simulink model "Parallel_n49"  (R2012b)
settings: Solver=VariableStepDiscrete  StartTime=0.0  StopTime=TotalIterations  RelTol=1e-3
values from neighbouring files (symbols this model uses):
  bp = 12    [ConfigValidate.m]
  bpSNMemory = bp    (= 12)    [ConfigValidate.m]
  IterationsOrdering = 4000    [ConfigValidate.m]
  MaxCoordDistance = (abs(max(wx) - min(wx))+abs(max(wy) - min(wy)))^2    [ConfigValidate.m]
  N_limit = 0.01    [ConfigValidate.m]
  nBits = 9    [ConfigValidate.m]
  nBitsNSmemories = (ceil(log2(TotalIterations)))    [ConfigValidate.m]
  S_limit = 1    [ConfigValidate.m]
  SourceNodes = 2000    [ConfigValidate.m]
  ts = 1    [ConfigValidate.m]
  w1 = rand(1,Neurons)    [ConfigValidate.m]
  w2 = rand(1,Neurons)    [ConfigValidate.m]
  wx = zeros(1,Neurons)    [ConfigValidate.m]
  wy = zeros(1,Neurons)    [ConfigValidate.m]
  x1 = rand(SourceNodes,1)    [ConfigValidate.m]
  x2 = rand(SourceNodes,1)    [ConfigValidate.m]
libraries: xbsIndex_r4 x4147, dspsrcs4 x2, dspstat3 x2
(part 1 of 19)
settings Model: Creator=Leonardo  LastModifiedBy=leona

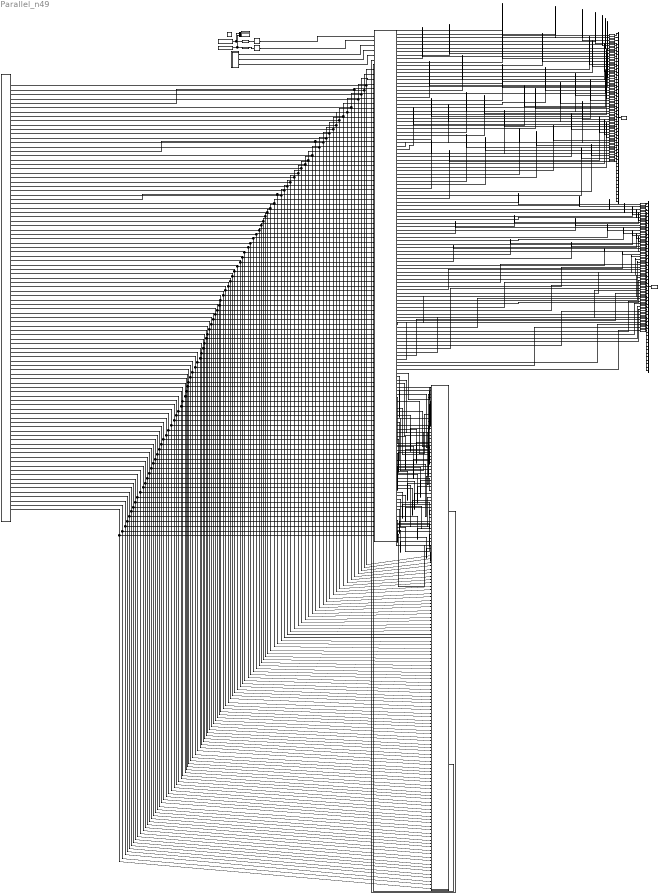
== system Parallel_n49 ==
  " System Generator" : xbsIndex_r4/ System Generator  Tag=genX  xilinxfamily=virtex6  part=xc6vlx240t  speed=-1  package=ff1156  synthesis_tool=XST  clock_wrapper=Clock Enables  directory=./n49d2nt  proj_type=Project Navigator  Synth_file=XST Defaults  Impl_file=ISE Defaults  testbench=off  simulink_period=ts  sysclk_period=10  dcm_input_clock_period=10  incr_netlist=off  trim_vbits=Everywhere in SubSystem  dbl_ovrd=According to Block Masks  core_generation=According to Block Masks  run_coregen=off  deprecated_control=off  eval_field=0  block_type=sysgen
  Coordinates : Subsystem
  Display2 : Display
  Gateway Out{1,3..48,53,65..75,77..107,109,113,120,126..128} (96 alike) : xbsIndex_r4/Gateway Out  inherit_from_input=off  hdl_port=off  timing_constraint=None  locs_specified=off  LOCs={}  UseAsDAC=off  DACChannel='1'  block_type=gatewayout
  Gateway Out2 : xbsIndex_r4/Gateway Out  inherit_from_input=off  hdl_port=on  timing_constraint=None  locs_specified=off  LOCs={}  UseAsDAC=off  DACChannel='1'  block_type=gatewayout
  Gateway Out76 : xbsIndex_r4/Gateway Out  inherit_from_input=off  hdl_port=on  timing_constraint=None  locs_specified=off  LOCs={}  UseAsDAC=off  DACChannel='1'  block_type=gatewayout
  Mux1 : Mux  Inputs=49
  Mux3 : Mux  Inputs=2
  Mux5 : Mux  Inputs=49
  Neurons : Subsystem
  Signal From Workspace : dspsrcs4/Signal From Workspace  X=x1(1:SourceNodes)  Ts=ts  nsamps=1  OutputAfterFinalValue=Cyclic repetition  ignoreOrWarnInputAndFrameLengths=off
  Signal From Workspace1 : dspsrcs4/Signal From Workspace  X=x2(1:SourceNodes)  Ts=ts  nsamps=1  OutputAfterFinalValue=Cyclic repetition  ignoreOrWarnInputAndFrameLengths=off
  TimeSeries_Functions : Subsystem
  To Workspace : ToWorkspace  VariableName=w1_histH  SampleTime=ts
  To Workspace1 : ToWorkspace  VariableName=w2_histH  SampleTime=ts
  WiningNeuronFinder1 : Subsystem
  delay_vX11 : xbsIndex_r4/Register  init=x1(1)  rst=off  en=off  dbl_ovrd=off  block_type=register
  delay_vX12 : xbsIndex_r4/Register  init=x2(1)  rst=off  en=off  dbl_ovrd=off  block_type=register
  "vX11_in " : xbsIndex_r4/Gateway In  gui_display_data_type=Fixed-point  arith_type="Signed  (2's comp)"  n_bits=nb  bin_pt=bp  preci_type=Single  exp_width=8  frac_width=24  quantization="Round  (unbiased: +/- Inf)"  overflow=Saturate  period=ts  dbl_ovrd=off  timing_constraint=None  locs_specified=off  LOCs={}  UseAsADC=off  ADCChannel='1'  inherit_from_input=off  hdl_port=on  block_type=gatewayin
  vX12_in : xbsIndex_r4/Gateway In  gui_display_data_type=Fixed-point  arith_type="Signed  (2's comp)"  n_bits=nb  bin_pt=bp  preci_type=Single  exp_width=8  frac_width=24  quantization="Round  (unbiased: +/- Inf)"  overflow=Saturate  period=ts  dbl_ovrd=off  timing_constraint=None  locs_specified=off  LOCs={}  UseAsADC=off  ADCChannel='1'  inherit_from_input=off  hdl_port=on  block_type=gatewayin
  wires:
  Signal From Workspace/1 -> Mux3/1, "vX11_in "/1
  Signal From Workspace1/1 -> Mux3/2, vX12_in/1
  Mux3/1 -> Display2/1
  vX12_in/1 -> delay_vX12/1
  delay_vX12/1 -> Neurons/2(vX12)
  TimeSeries_Functions/1(S) -> Neurons/3(S)
  TimeSeries_Functions/2(N) -> Neurons/4(N)
  TimeSeries_Functions/3(MemControl) -> Neurons/5(memControl)
  Mux5/1 -> To Workspace/1
  "vX11_in "/1 -> delay_vX11/1
  delay_vX11/1 -> Neurons/1(vX11)
  Neurons/34(w1n34) -> Gateway Out27/1
  Neurons/35(w1n35) -> Gateway Out26/1
  Neurons/31(w1n31) -> Gateway Out35/1
  Neurons/33(w1n33) -> Gateway Out36/1
  Neurons/32(w1n32) -> Gateway Out34/1
  Neurons/40(w1n40) -> Gateway Out44/1
  Neurons/45(w1n45) -> Gateway Out48/1
  Neurons/36(w1n36) -> Gateway Out28/1
  Neurons/44(w1n44) -> Gateway Out46/1
  Neurons/39(w1n39) -> Gateway Out42/1
  Neurons/43(w1n43) -> Gateway Out47/1
  Neurons/42(w1n42) -> Gateway Out45/1
  Neurons/37(w1n37) -> Gateway Out41/1
  Neurons/38(w1n38) -> Gateway Out37/1
  Neurons/41(w1n41) -> Gateway Out43/1
  Neurons/27(w1n27) -> Gateway Out30/1
  Neurons/26(w1n26) -> Gateway Out25/1
  Neurons/29(w1n29) -> Gateway Out31/1
  Neurons/28(w1n28) -> Gateway Out32/1
  Neurons/30(w1n30) -> Gateway Out33/1
  Neurons/6(w1n6) -> Gateway Out6/1
  Neurons/9(w1n9) -> Gateway Out9/1
  Neurons/10(w1n10) -> Gateway Out11/1
  Neurons/1(w1n1) -> Gateway Out2/1
  Neurons/2(w1n2) -> Gateway Out1/1
  Neurons/3(w1n3) -> Gateway Out3/1
  Neurons/4(w1n4) -> Gateway Out5/1
  Neurons/5(w1n5) -> Gateway Out4/1
  Neurons/7(w1n7) -> Gateway Out8/1
  Neurons/8(w1n8) -> Gateway Out7/1
  Neurons/23(w1n23) -> Gateway Out14/1
  Neurons/12(w1n12) -> Gateway Out12/1
  Neurons/11(w1n11) -> Gateway Out10/1
  Neurons/14(w1n14) -> Gateway Out13/1
  Neurons/19(w1n19) -> Gateway Out23/1
  Neurons/24(w1n24) -> Gateway Out16/1
  Neurons/13(w1n13) -> Gateway Out17/1
  Neurons/15(w1n15) -> Gateway Out18/1
  Neurons/18(w1n18) -> Gateway Out21/1
  Neurons/17(w1n17) -> Gateway Out19/1
  Neurons/20(w1n20) -> Gateway Out22/1
  Neurons/22(w1n22) -> Gateway Out15/1
  Neurons/25(w1n25) -> Gateway Out29/1
  Neurons/16(w1n16) -> Gateway Out20/1
  Neurons/21(w1n21) -> Gateway Out24/1
  Neurons/48(w1n48) -> Gateway Out40/1
  Neurons/46(w1n46) -> Gateway Out39/1
  Neurons/49(w1n49) -> Gateway Out53/1
  Neurons/47(w1n47) -> Gateway Out38/1
  Mux1/1 -> To Workspace1/1
  Neurons/70(w2n21) -> Gateway Out81/1
  Neurons/72(w2n23) -> Gateway Out70/1
  Neurons/71(w2n22) -> Gateway Out71/1
  Neurons/74(w2n25) -> Gateway Out86/1
  Neurons/73(w2n24) -> Gateway Out72/1
  Neurons/60(w2n11) -> Gateway Out66/1
  Neurons/63(w2n14) -> Gateway Out69/1
  Neurons/62(w2n13) -> Gateway Out73/1
  Neurons/64(w2n15) -> Gateway Out74/1
  Neurons/61(w2n12) -> Gateway Out68/1
  Neurons/54(w2n5) -> Gateway Out98/1
  Neurons/85(w2n36) -> Gateway Out85/1
  Neurons/88(w2n39) -> Gateway Out101/1
  Neurons/89(w2n40) -> Gateway Out103/1
  Neurons/86(w2n37) -> Gateway Out100/1
  Neurons/87(w2n38) -> Gateway Out95/1
  Neurons/94(w2n45) -> Gateway Out107/1
  Neurons/93(w2n44) -> Gateway Out105/1
  Neurons/92(w2n43) -> Gateway Out106/1
  Neurons/90(w2n41) -> Gateway Out102/1
  Neurons/91(w2n42) -> Gateway Out104/1
  Neurons/65(w2n16) -> Gateway Out77/1
  Neurons/68(w2n19) -> Gateway Out80/1
  Neurons/67(w2n18) -> Gateway Out78/1
  Neurons/66(w2n17) -> Gateway Out75/1
  Neurons/69(w2n20) -> Gateway Out79/1
  Neurons/55(w2n6) -> Gateway Out120/1
  Neurons/56(w2n7) -> Gateway Out127/1
  Neurons/59(w2n10) -> Gateway Out67/1
  Neurons/57(w2n8) -> Gateway Out126/1
  Neurons/58(w2n9) -> Gateway Out128/1
  Neurons/75(w2n26) -> Gateway Out82/1
  Neurons/78(w2n29) -> Gateway Out89/1
  Neurons/79(w2n30) -> Gateway Out91/1
  Neurons/76(w2n27) -> Gateway Out88/1
  Neurons/77(w2n28) -> Gateway Out90/1
  Neurons/52(w2n3) -> Gateway Out87/1
  Neurons/95(w2n46) -> Gateway Out97/1
  Neurons/97(w2n48) -> Gateway Out99/1
  Neurons/96(w2n47) -> Gateway Out96/1
  Neurons/98(w2n49) -> Gateway Out113/1
  Neurons/51(w2n2) -> Gateway Out65/1
  Neurons/50(w2n1) -> Gateway Out76/1
  Neurons/80(w2n31) -> Gateway Out93/1
  Neurons/81(w2n32) -> Gateway Out92/1
  Neurons/82(w2n33) -> Gateway Out94/1
  Neurons/84(w2n35) -> Gateway Out83/1
  Neurons/83(w2n34) -> Gateway Out84/1
  Neurons/53(w2n4) -> Gateway Out109/1
  Gateway Out2/1 -> Mux5/1
  Gateway Out1/1 -> Mux5/2
  Gateway Out3/1 -> Mux5/3
  Gateway Out5/1 -> Mux5/4
  Gateway Out6/1 -> Mux5/6
  Gateway Out4/1 -> Mux5/5
  Gateway Out8/1 -> Mux5/7
  Gateway Out10/1 -> Mux5/11
  Gateway Out9/1 -> Mux5/9
  Gateway Out7/1 -> Mux5/8
  Gateway Out11/1 -> Mux5/10
  Gateway Out12/1 -> Mux5/12
  Gateway Out13/1 -> Mux5/14
  Gateway Out22/1 -> Mux5/20
  Gateway Out17/1 -> Mux5/13
  Gateway Out20/1 -> Mux5/16
  Gateway Out14/1 -> Mux5/23
  Gateway Out15/1 -> Mux5/22
  Gateway Out16/1 -> Mux5/24
  Gateway Out19/1 -> Mux5/17
  Gateway Out18/1 -> Mux5/15
  Gateway Out21/1 -> Mux5/18
  Gateway Out23/1 -> Mux5/19
  Gateway Out24/1 -> Mux5/21
  Gateway Out25/1 -> Mux5/26
  Gateway Out27/1 -> Mux5/34
  Gateway Out26/1 -> Mux5/35
  Gateway Out28/1 -> Mux5/36
  Gateway Out36/1 -> Mux5/33
  Gateway Out30/1 -> Mux5/27
  Gateway Out32/1 -> Mux5/28
  Gateway Out29/1 -> Mux5/25
  Gateway Out35/1 -> Mux5/31
  Gateway Out31/1 -> Mux5/29
  Gateway Out34/1 -> Mux5/32
  Gateway Out33/1 -> Mux5/30
  Gateway Out45/1 -> Mux5/42
  Gateway Out43/1 -> Mux5/41
  Gateway Out44/1 -> Mux5/40
  Gateway Out46/1 -> Mux5/44
  Gateway Out39/1 -> Mux5/46
  Gateway Out41/1 -> Mux5/37
  Gateway Out40/1 -> Mux5/48
  Gateway Out38/1 -> Mux5/47
  Gateway Out42/1 -> Mux5/39
  Gateway Out37/1 -> Mux5/38
  Gateway Out48/1 -> Mux5/45
  Gateway Out47/1 -> Mux5/43
  Gateway Out53/1 -> Mux5/49
  Gateway Out66/1 -> Mux1/11
  Gateway Out69/1 -> Mux1/14
  Gateway Out67/1 -> Mux1/10
  Gateway Out70/1 -> Mux1/23
  Gateway Out68/1 -> Mux1/12
  Gateway Out73/1 -> Mux1/13
  Gateway Out72/1 -> Mux1/24
  Gateway Out75/1 -> Mux1/17
  Gateway Out71/1 -> Mux1/22
  Gateway Out74/1 -> Mux1/15
  Gateway Out79/1 -> Mux1/20
  Gateway Out80/1 -> Mux1/19
  Gateway Out76/1 -> Mux1/1
  Gateway Out77/1 -> Mux1/16
  Gateway Out78/1 -> Mux1/18
  Gateway Out84/1 -> Mux1/34
  Gateway Out85/1 -> Mux1/36
  Gateway Out82/1 -> Mux1/26
  Gateway Out81/1 -> Mux1/21
  Gateway Out83/1 -> Mux1/35
  Gateway Out88/1 -> Mux1/27
  Gateway Out90/1 -> Mux1/28
  Gateway Out89/1 -> Mux1/29
  Gateway Out86/1 -> Mux1/25
  Gateway Out87/1 -> Mux1/3
  Gateway Out92/1 -> Mux1/32
  Gateway Out93/1 -> Mux1/31
  Gateway Out94/1 -> Mux1/33
  Gateway Out91/1 -> Mux1/30
  Gateway Out95/1 -> Mux1/38
  Gateway Out96/1 -> Mux1/47
  Gateway Out98/1 -> Mux1/5
  Gateway Out97/1 -> Mux1/46
  Gateway Out99/1 -> Mux1/48
  Gateway Out101/1 -> Mux1/39
  Gateway Out100/1 -> Mux1/37
  Gateway Out65/1 -> Mux1/2
  Gateway Out102/1 -> Mux1/41
  Gateway Out113/1 -> Mux1/49
  Gateway Out106/1 -> Mux1/43
  Gateway Out105/1 -> Mux1/44
  Gateway Out104/1 -> Mux1/42
  Gateway Out109/1 -> Mux1/4
  Gateway Out107/1 -> Mux1/45
  Gateway Out103/1 -> Mux1/40
  Gateway Out127/1 -> Mux1/7
  Gateway Out128/1 -> Mux1/9
  Gateway Out120/1 -> Mux1/6
  Gateway Out126/1 -> Mux1/8
  Neurons/109(dist_n11) -> WiningNeuronFinder1/11(dist_k11)
  Neurons/113(dist_n15) -> WiningNeuronFinder1/15(dist_k15)
  Neurons/112(dist_n14) -> WiningNeuronFinder1/14(dist_k14)
  Neurons/110(dist_n12) -> WiningNeuronFinder1/12(dist_k12)
  Neurons/111(dist_n13) -> WiningNeuronFinder1/13(dist_k13)
  Neurons/120(dist_n22) -> WiningNeuronFinder1/22(dist_k22)
  Neurons/123(dist_n25) -> WiningNeuronFinder1/25(dist_k25)
  Neurons/122(dist_n24) -> WiningNeuronFinder1/24(dist_k24)
  Neurons/121(dist_n23) -> WiningNeuronFinder1/23(dist_k23)
  Neurons/119(dist_n21) -> WiningNeuronFinder1/21(dist_k21)
  Neurons/114(dist_n16) -> WiningNeuronFinder1/16(dist_k16)
  Neurons/115(dist_n17) -> WiningNeuronFinder1/17(dist_k17)
  Neurons/118(dist_n20) -> WiningNeuronFinder1/20(dist_k20)
  Neurons/117(dist_n19) -> WiningNeuronFinder1/19(dist_k19)
  Neurons/116(dist_n18) -> WiningNeuronFinder1/18(dist_k18)
  Neurons/99(dist_n1) -> WiningNeuronFinder1/1(dist_k1)
  Neurons/139(dist_n41) -> WiningNeuronFinder1/41(dist_k41)
  Neurons/142(dist_n44) -> WiningNeuronFinder1/44(dist_k44)
  Neurons/141(dist_n43) -> WiningNeuronFinder1/43(dist_k43)
  Neurons/143(dist_n45) -> WiningNeuronFinder1/45(dist_k45)
  Neurons/140(dist_n42) -> WiningNeuronFinder1/42(dist_k42)
  Neurons/145(dist_n47) -> WiningNeuronFinder1/47(dist_k47)
  Neurons/144(dist_n46) -> WiningNeuronFinder1/46(dist_k46)
  Neurons/146(dist_n48) -> WiningNeuronFinder1/48(dist_k48)
  Neurons/147(dist_n49) -> WiningNeuronFinder1/49(dist_k49)
  Neurons/101(dist_n3) -> WiningNeuronFinder1/3(dist_k3)
  Neurons/102(dist_n4) -> WiningNeuronFinder1/4(dist_k4)
  Neurons/125(dist_n27) -> WiningNeuronFinder1/27(dist_k27)
  Neurons/126(dist_n28) -> WiningNeuronFinder1/28(dist_k28)
  Neurons/127(dist_n29) -> WiningNeuronFinder1/29(dist_k29)
  Neurons/128(dist_n30) -> WiningNeuronFinder1/30(dist_k30)
  Neurons/124(dist_n26) -> WiningNeuronFinder1/26(dist_k26)
  Neurons/100(dist_n2) -> WiningNeuronFinder1/2(dist_k2)
  Neurons/129(dist_n31) -> WiningNeuronFinder1/31(dist_k31)
  Neurons/133(dist_n35) -> WiningNeuronFinder1/35(dist_k35)
  Neurons/131(dist_n33) -> WiningNeuronFinder1/33(dist_k33)
  Neurons/130(dist_n32) -> WiningNeuronFinder1/32(dist_k32)
  Neurons/132(dist_n34) -> WiningNeuronFinder1/34(dist_k34)
  Neurons/138(dist_n40) -> WiningNeuronFinder1/40(dist_k40)
  Neurons/136(dist_n38) -> WiningNeuronFinder1/38(dist_k38)
  Neurons/135(dist_n37) -> WiningNeuronFinder1/37(dist_k37)
  Neurons/134(dist_n36) -> WiningNeuronFinder1/36(dist_k36)
  Neurons/137(dist_n39) -> WiningNeuronFinder1/39(dist_k39)
  Neurons/103(dist_n5) -> WiningNeuronFinder1/5(dist_k5)
  Neurons/108(dist_n10) -> WiningNeuronFinder1/10(dist_k10)
  Neurons/107(dist_n9) -> WiningNeuronFinder1/9(dist_k9)
  Neurons/104(dist_n6) -> WiningNeuronFinder1/6(dist_k6)
  Neurons/106(dist_n8) -> WiningNeuronFinder1/8(dist_k8)
  Neurons/105(dist_n7) -> WiningNeuronFinder1/7(dist_k7)
  WiningNeuronFinder1/1(WinningNeuron_wx) -> Neurons/6(wx_win)
  WiningNeuronFinder1/2(WinningNeuron_wy) -> Neurons/7(wy_win)
  Coordinates/98(wy49) -> WiningNeuronFinder1/147(wy_49), Neurons/105(wy49)
  Coordinates/97(wx49) -> WiningNeuronFinder1/146(wx_49), Neurons/104(wx49)
  Coordinates/96(wy48) -> WiningNeuronFinder1/145(wy_48), Neurons/103(wy48)
  Coordinates/95(wx48) -> WiningNeuronFinder1/144(wx_48), Neurons/102(wx48)
  Coordinates/93(wx47) -> WiningNeuronFinder1/142(wx_47), Neurons/100(wx47)
  Coordinates/92(wy46) -> WiningNeuronFinder1/141(wy_46), Neurons/99(wy46)
  Coordinates/91(wx46) -> WiningNeuronFinder1/140(wx_46), Neurons/98(wx46)
  Coordinates/90(wy45) -> WiningNeuronFinder1/139(wy_45), Neurons/97(wy45)
  Coordinates/88(wy44) -> WiningNeuronFinder1/137(wy_44), Neurons/95(wy44)
  Coordinates/87(wx44) -> WiningNeuronFinder1/136(wx_44), Neurons/94(wx44)
  Coordinates/86(wy43) -> WiningNeuronFinder1/135(wy_43), Neurons/93(wy43)
  Coordinates/85(wx43) -> WiningNeuronFinder1/134(wx_43), Neurons/92(wx43)
  Coordinates/84(wy42) -> WiningNeuronFinder1/133(wy_42), Neurons/91(wy42)
  Coordinates/83(wx42) -> WiningNeuronFinder1/132(wx_42), Neurons/90(wx42)
  Coordinates/81(wx41) -> WiningNeuronFinder1/130(wx_41), Neurons/88(wx41)
  Coordinates/80(wy40) -> WiningNeuronFinder1/129(wy_40), Neurons/87(wy40)
  Coordinates/79(wx40) -> WiningNeuronFinder1/128(wx_40), Neurons/86(wx40)
  Coordinates/78(wy39) -> WiningNeuronFinder1/127(wy_39), Neurons/85(wy39)
  Coordinates/77(wx39) -> WiningNeuronFinder1/126(wx_39), Neurons/84(wx39)
  Coordinates/76(wy38) -> WiningNeuronFinder1/125(wy_38), Neurons/83(wy38)
  Coordinates/75(wx38) -> WiningNeuronFinder1/124(wx_38), Neurons/82(wx38)
  Coordinates/74(wy37) -> WiningNeuronFinder1/123(wy_37), Neurons/81(wy37)
  Coordinates/73(wx37) -> WiningNeuronFinder1/122(wx_37), Neurons/80(wx37)
  Coordinates/72(wy36) -> WiningNeuronFinder1/121(wy_36), Neurons/79(wy36)
  Coordinates/71(wx36) -> WiningNeuronFinder1/120(wx_36), Neurons/78(wx36)
  Coordinates/70(wy35) -> WiningNeuronFinder1/119(wy_35), Neurons/77(wy35)
  Coordinates/69(wx35) -> WiningNeuronFinder1/118(wx_35), Neurons/76(wx35)
  Coordinates/68(wy34) -> WiningNeuronFinder1/117(wy_34), Neurons/75(wy34)
  Coordinates/67(wx34) -> WiningNeuronFinder1/116(wx_34), Neurons/74(wx34)
  Coordinates/66(wy33) -> WiningNeuronFinder1/115(wy_33), Neurons/73(wy33)
  Coordinates/65(wx33) -> WiningNeuronFinder1/114(wx_33), Neurons/72(wx33)
  Coordinates/63(wx32) -> WiningNeuronFinder1/112(wx_32), Neurons/70(wx32)
  Coordinates/62(wy31) -> WiningNeuronFinder1/111(wy_31), Neurons/69(wy31)
  Coordinates/61(wx31) -> WiningNeuronFinder1/110(wx_31), Neurons/68(wx31)
  Coordinates/59(wx30) -> WiningNeuronFinder1/108(wx_30), Neurons/66(wx30)
  Coordinates/58(wy29) -> WiningNeuronFinder1/107(wy_29), Neurons/65(wy29)
  Coordinates/57(wx29) -> WiningNeuronFinder1/106(wx_29), Neurons/64(wx29)
  Coordinates/56(wy28) -> WiningNeuronFinder1/105(wy_28), Neurons/63(wy28)
  Coordinates/54(wy27) -> WiningNeuronFinder1/103(wy_27), Neurons/61(wy27)
  Coordinates/53(wx27) -> WiningNeuronFinder1/102(wx_27), Neurons/60(wx27)
  Coordinates/52(wy26) -> WiningNeuronFinder1/101(wy_26), Neurons/59(wy26)
  Coordinates/51(wx26) -> WiningNeuronFinder1/100(wx_26), Neurons/58(wx26)
  Coordinates/50(wy25) -> WiningNeuronFinder1/99(wy_25), Neurons/57(wy25)
  Coordinates/49(wx25) -> WiningNeuronFinder1/98(wx_25), Neurons/56(wx25)
  Coordinates/48(wy24) -> WiningNeuronFinder1/97(wy_24), Neurons/55(wy24)
  Coordinates/47(wx24) -> WiningNeuronFinder1/96(wx_24), Neurons/54(wx24)
  Coordinates/46(wy23) -> WiningNeuronFinder1/95(wy_23), Neurons/53(wy23)
  Coordinates/45(wx23) -> WiningNeuronFinder1/94(wx_23), Neurons/52(wx23)
  Coordinates/43(wx22) -> WiningNeuronFinder1/92(wx_22), Neurons/50(wx22)
  Coordinates/42(wy21) -> WiningNeuronFinder1/91(wy_21), Neurons/49(wy21)
  Coordinates/41(wx21) -> WiningNeuronFinder1/90(wx_21), Neurons/48(wx21)
  Coordinates/40(wy20) -> WiningNeuronFinder1/89(wy_20), Neurons/47(wy20)
  Coordinates/39(wx20) -> WiningNeuronFinder1/88(wx_20), Neurons/46(wx20)
  Coordinates/38(wy19) -> WiningNeuronFinder1/87(wy_19), Neurons/45(wy19)
  Coordinates/37(wx19) -> WiningNeuronFinder1/86(wx_19), Neurons/44(wx19)
  Coordinates/36(wy18) -> WiningNeuronFinder1/85(wy_18), Neurons/43(wy18)
  Coordinates/35(wx18) -> WiningNeuronFinder1/84(wx_18), Neurons/42(wx18)
  Coordinates/34(wy17) -> WiningNeuronFinder1/83(wy_17), Neurons/41(wy17)
  Coordinates/32(wy16) -> WiningNeuronFinder1/81(wy_16), Neurons/39(wy16)
  Coordinates/31(wx16) -> WiningNeuronFinder1/80(wx_16), Neurons/38(wx16)
  Coordinates/30(wy15) -> WiningNeuronFinder1/79(wy_15), Neurons/37(wy15)
  Coordinates/29(wx15) -> WiningNeuronFinder1/78(wx_15), Neurons/36(wx15)
  Coordinates/28(wy14) -> WiningNeuronFinder1/77(wy_14), Neurons/35(wy14)
  Coordinates/27(wx14) -> WiningNeuronFinder1/76(wx_14), Neurons/34(wx14)
  Coordinates/26(wy13) -> WiningNeuronFinder1/75(wy_13), Neurons/33(wy13)
  Coordinates/25(wx13) -> WiningNeuronFinder1/74(wx_13), Neurons/32(wx13)
  Coordinates/23(wx12) -> WiningNeuronFinder1/72(wx_12), Neurons/30(wx12)
  Coordinates/22(wy11) -> WiningNeuronFinder1/71(wy_11), Neurons/29(wy11)
  Coordinates/21(wx11) -> WiningNeuronFinder1/70(wx_11), Neurons/28(wx11)
  Coordinates/20(wy10) -> WiningNeuronFinder1/69(wy_10), Neurons/27(wy10)
  Coordinates/19(wx10) -> WiningNeuronFinder1/68(wx_10), Neurons/26(wx10)
  Coordinates/18(wy9) -> WiningNeuronFinder1/67(wy_9), Neurons/25(wy9)
  Coordinates/17(wx9) -> WiningNeuronFinder1/66(wx_9), Neurons/24(wx9)
  Coordinates/16(wy8) -> WiningNeuronFinder1/65(wy_8), Neurons/23(wy8)
  Coordinates/15(wx8) -> WiningNeuronFinder1/64(wx_8), Neurons/22(wx8)
  Coordinates/14(wy7) -> WiningNeuronFinder1/63(wy_7), Neurons/21(wy7)
  Coordinates/13(wx7) -> WiningNeuronFinder1/62(wx_7), Neurons/20(wx7)
  Coordinates/12(wy6) -> WiningNeuronFinder1/61(wy_6), Neurons/19(wy6)
  Coordinates/11(wx6) -> WiningNeuronFinder1/60(wx_6), Neurons/18(wx6)
  Coordinates/10(wy5) -> WiningNeuronFinder1/59(wy_5), Neurons/17(wy5)
  Coordinates/9(wx5) -> WiningNeuronFinder1/58(wx_5), Neurons/16(wx5)
  Coordinates/8(wy4) -> WiningNeuronFinder1/57(wy_4), Neurons/15(wy4)
  Coordinates/7(wx4) -> WiningNeuronFinder1/56(wx_4), Neurons/14(wx4)
  Coordinates/6(wy3) -> WiningNeuronFinder1/55(wy_3), Neurons/13(wy3)
  Coordinates/4(wy2) -> WiningNeuronFinder1/53(wy_2), Neurons/11(wy2)
  Coordinates/2(wy1) -> WiningNeuronFinder1/51(wy_1), Neurons/9(wy1)
  Coordinates/1(wx1) -> WiningNeuronFinder1/50(wx_1), Neurons/8(wx1)
  Coordinates/3(wx2) -> WiningNeuronFinder1/52(wx_2), Neurons/10(wx2)
  Coordinates/5(wx3) -> WiningNeuronFinder1/54(wx_3), Neurons/12(wx3)
  Coordinates/24(wy12) -> WiningNeuronFinder1/73(wy_12), Neurons/31(wy12)
  Coordinates/33(wx17) -> WiningNeuronFinder1/82(wx_17), Neurons/40(wx17)
  Coordinates/44(wy22) -> WiningNeuronFinder1/93(wy_22), Neurons/51(wy22)
  Coordinates/55(wx28) -> WiningNeuronFinder1/104(wx_28), Neurons/62(wx28)
  Coordinates/60(wy30) -> WiningNeuronFinder1/109(wy_30), Neurons/67(wy30)
  Coordinates/64(wy32) -> WiningNeuronFinder1/113(wy_32), Neurons/71(wy32)
  Coordinates/82(wy41) -> WiningNeuronFinder1/131(wy_41), Neurons/89(wy41)
  Coordinates/89(wx45) -> WiningNeuronFinder1/138(wx_45), Neurons/96(wx45)
  Coordinates/94(wy47) -> WiningNeuronFinder1/143(wy_47), Neurons/101(wy47)

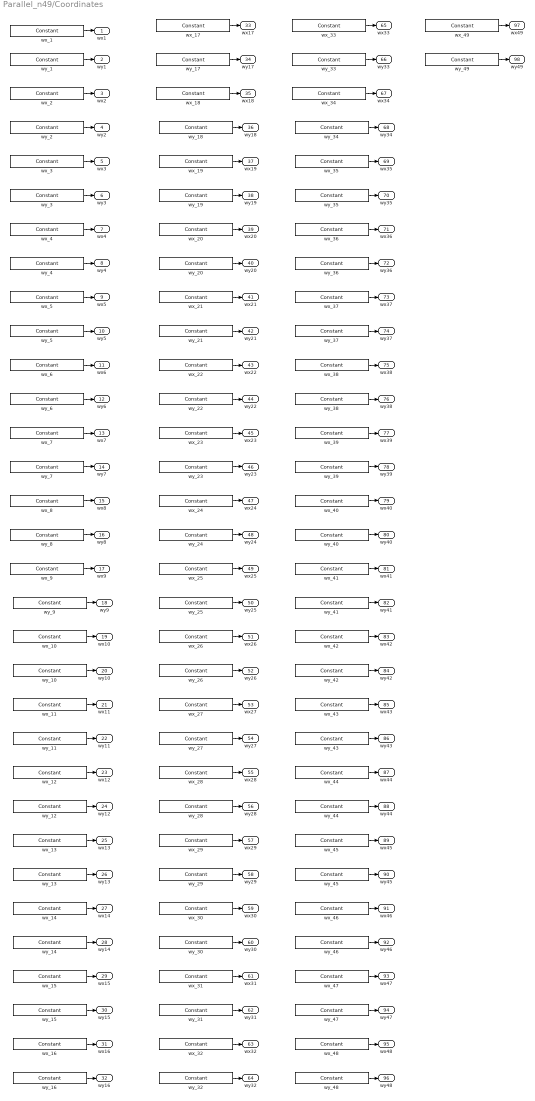
== system Parallel_n49/Coordinates ==
  wx_1 : xbsIndex_r4/Constant  const=wx(1)  gui_display_data_type=Fixed-point  arith_type=Unsigned  n_bits=nbCoord  bin_pt=bpCoord  preci_type=Single  exp_width=8  frac_width=24  explicit_period=on  period=ts  equ=P=C  opselect=C  inp2=PCIN>>17  opr=+  inp1=P  carry=CIN  dbl_ovrd=off  block_type=constant
  wx_10 : xbsIndex_r4/Constant  const=wx(10)  gui_display_data_type=Fixed-point  arith_type=Unsigned  n_bits=nbCoord  bin_pt=bpCoord  preci_type=Single  exp_width=8  frac_width=24  explicit_period=on  period=ts  equ=P=C  opselect=C  inp2=PCIN>>17  opr=+  inp1=P  carry=CIN  dbl_ovrd=off  block_type=constant
  wx_11 : xbsIndex_r4/Constant  const=wx(11)  gui_display_data_type=Fixed-point  arith_type=Unsigned  n_bits=nbCoord  bin_pt=bpCoord  preci_type=Single  exp_width=8  frac_width=24  explicit_period=on  period=ts  equ=P=C  opselect=C  inp2=PCIN>>17  opr=+  inp1=P  carry=CIN  dbl_ovrd=off  block_type=constant
  wx_12 : xbsIndex_r4/Constant  const=wx(12)  gui_display_data_type=Fixed-point  arith_type=Unsigned  n_bits=nbCoord  bin_pt=bpCoord  preci_type=Single  exp_width=8  frac_width=24  explicit_period=on  period=ts  equ=P=C  opselect=C  inp2=PCIN>>17  opr=+  inp1=P  carry=CIN  dbl_ovrd=off  block_type=constant
  wx_13 : xbsIndex_r4/Constant  const=wx(13)  gui_display_data_type=Fixed-point  arith_type=Unsigned  n_bits=nbCoord  bin_pt=bpCoord  preci_type=Single  exp_width=8  frac_width=24  explicit_period=on  period=ts  equ=P=C  opselect=C  inp2=PCIN>>17  opr=+  inp1=P  carry=CIN  dbl_ovrd=off  block_type=constant
  wx_14 : xbsIndex_r4/Constant  const=wx(14)  gui_display_data_type=Fixed-point  arith_type=Unsigned  n_bits=nbCoord  bin_pt=bpCoord  preci_type=Single  exp_width=8  frac_width=24  explicit_period=on  period=ts  equ=P=C  opselect=C  inp2=PCIN>>17  opr=+  inp1=P  carry=CIN  dbl_ovrd=off  block_type=constant
  wx_15 : xbsIndex_r4/Constant  const=wx(15)  gui_display_data_type=Fixed-point  arith_type=Unsigned  n_bits=nbCoord  bin_pt=bpCoord  preci_type=Single  exp_width=8  frac_width=24  explicit_period=on  period=ts  equ=P=C  opselect=C  inp2=PCIN>>17  opr=+  inp1=P  carry=CIN  dbl_ovrd=off  block_type=constant
  wx_16 : xbsIndex_r4/Constant  const=wx(16)  gui_display_data_type=Fixed-point  arith_type=Unsigned  n_bits=nbCoord  bin_pt=bpCoord  preci_type=Single  exp_width=8  frac_width=24  explicit_period=on  period=ts  equ=P=C  opselect=C  inp2=PCIN>>17  opr=+  inp1=P  carry=CIN  dbl_ovrd=off  block_type=constant
  wx_17 : xbsIndex_r4/Constant  const=wx(17)  gui_display_data_type=Fixed-point  arith_type=Unsigned  n_bits=nbCoord  bin_pt=bpCoord  preci_type=Single  exp_width=8  frac_width=24  explicit_period=on  period=ts  equ=P=C  opselect=C  inp2=PCIN>>17  opr=+  inp1=P  carry=CIN  dbl_ovrd=off  block_type=constant
  wx_18 : xbsIndex_r4/Constant  const=wx(18)  gui_display_data_type=Fixed-point  arith_type=Unsigned  n_bits=nbCoord  bin_pt=bpCoord  preci_type=Single  exp_width=8  frac_width=24  explicit_period=on  period=ts  equ=P=C  opselect=C  inp2=PCIN>>17  opr=+  inp1=P  carry=CIN  dbl_ovrd=off  block_type=constant
  wx_{19,26,35,42} (4 alike) : xbsIndex_r4/Constant  const=wx(19)  gui_display_data_type=Fixed-point  arith_type=Unsigned  n_bits=nbCoord  bin_pt=bpCoord  preci_type=Single  exp_width=8  frac_width=24  explicit_period=on  period=ts  equ=P=C  opselect=C  inp2=PCIN>>17  opr=+  inp1=P  carry=CIN  dbl_ovrd=off  block_type=constant
  wx_2 : xbsIndex_r4/Constant  const=wx(2)  gui_display_data_type=Fixed-point  arith_type=Unsigned  n_bits=nbCoord  bin_pt=bpCoord  preci_type=Single  exp_width=8  frac_width=24  explicit_period=on  period=ts  equ=P=C  opselect=C  inp2=PCIN>>17  opr=+  inp1=P  carry=CIN  dbl_ovrd=off  block_type=constant
  wx_{20,27,36,43} (4 alike) : xbsIndex_r4/Constant  const=wx(20)  gui_display_data_type=Fixed-point  arith_type=Unsigned  n_bits=nbCoord  bin_pt=bpCoord  preci_type=Single  exp_width=8  frac_width=24  explicit_period=on  period=ts  equ=P=C  opselect=C  inp2=PCIN>>17  opr=+  inp1=P  carry=CIN  dbl_ovrd=off  block_type=constant
  wx_{21,28,37,44} (4 alike) : xbsIndex_r4/Constant  const=wx(21)  gui_display_data_type=Fixed-point  arith_type=Unsigned  n_bits=nbCoord  bin_pt=bpCoord  preci_type=Single  exp_width=8  frac_width=24  explicit_period=on  period=ts  equ=P=C  opselect=C  inp2=PCIN>>17  opr=+  inp1=P  carry=CIN  dbl_ovrd=off  block_type=constant
  wx_{22,29,38,45} (4 alike) : xbsIndex_r4/Constant  const=wx(22)  gui_display_data_type=Fixed-point  arith_type=Unsigned  n_bits=nbCoord  bin_pt=bpCoord  preci_type=Single  exp_width=8  frac_width=24  explicit_period=on  period=ts  equ=P=C  opselect=C  inp2=PCIN>>17  opr=+  inp1=P  carry=CIN  dbl_ovrd=off  block_type=constant
  wx_{23,30,39,46} (4 alike) : xbsIndex_r4/Constant  const=wx(23)  gui_display_data_type=Fixed-point  arith_type=Unsigned  n_bits=nbCoord  bin_pt=bpCoord  preci_type=Single  exp_width=8  frac_width=24  explicit_period=on  period=ts  equ=P=C  opselect=C  inp2=PCIN>>17  opr=+  inp1=P  carry=CIN  dbl_ovrd=off  block_type=constant
  wx_{24,31,40,47} (4 alike) : xbsIndex_r4/Constant  const=wx(24)  gui_display_data_type=Fixed-point  arith_type=Unsigned  n_bits=nbCoord  bin_pt=bpCoord  preci_type=Single  exp_width=8  frac_width=24  explicit_period=on  period=ts  equ=P=C  opselect=C  inp2=PCIN>>17  opr=+  inp1=P  carry=CIN  dbl_ovrd=off  block_type=constant
  wx_{25,32,41,48} (4 alike) : xbsIndex_r4/Constant  const=wx(25)  gui_display_data_type=Fixed-point  arith_type=Unsigned  n_bits=nbCoord  bin_pt=bpCoord  preci_type=Single  exp_width=8  frac_width=24  explicit_period=on  period=ts  equ=P=C  opselect=C  inp2=PCIN>>17  opr=+  inp1=P  carry=CIN  dbl_ovrd=off  block_type=constant
  wx_3 : xbsIndex_r4/Constant  const=wx(3)  gui_display_data_type=Fixed-point  arith_type=Unsigned  n_bits=nbCoord  bin_pt=bpCoord  preci_type=Single  exp_width=8  frac_width=24  explicit_period=on  period=ts  equ=P=C  opselect=C  inp2=PCIN>>17  opr=+  inp1=P  carry=CIN  dbl_ovrd=off  block_type=constant
  wx_33 : xbsIndex_r4/Constant  const=wx(17)  gui_display_data_type=Fixed-point  arith_type=Unsigned  n_bits=nbCoord  bin_pt=bpCoord  preci_type=Single  exp_width=8  frac_width=24  explicit_period=on  period=ts  equ=P=C  opselect=C  inp2=PCIN>>17  opr=+  inp1=P  carry=CIN  dbl_ovrd=off  block_type=constant
  wx_34 : xbsIndex_r4/Constant  const=wx(18)  gui_display_data_type=Fixed-point  arith_type=Unsigned  n_bits=nbCoord  bin_pt=bpCoord  preci_type=Single  exp_width=8  frac_width=24  explicit_period=on  period=ts  equ=P=C  opselect=C  inp2=PCIN>>17  opr=+  inp1=P  carry=CIN  dbl_ovrd=off  block_type=constant
  wx_4 : xbsIndex_r4/Constant  const=wx(4)  gui_display_data_type=Fixed-point  arith_type=Unsigned  n_bits=nbCoord  bin_pt=bpCoord  preci_type=Single  exp_width=8  frac_width=24  explicit_period=on  period=ts  equ=P=C  opselect=C  inp2=PCIN>>17  opr=+  inp1=P  carry=CIN  dbl_ovrd=off  block_type=constant
  wx_49 : xbsIndex_r4/Constant  const=wx(17)  gui_display_data_type=Fixed-point  arith_type=Unsigned  n_bits=nbCoord  bin_pt=bpCoord  preci_type=Single  exp_width=8  frac_width=24  explicit_period=on  period=ts  equ=P=C  opselect=C  inp2=PCIN>>17  opr=+  inp1=P  carry=CIN  dbl_ovrd=off  block_type=constant
  wx_5 : xbsIndex_r4/Constant  const=wx(5)  gui_display_data_type=Fixed-point  arith_type=Unsigned  n_bits=nbCoord  bin_pt=bpCoord  preci_type=Single  exp_width=8  frac_width=24  explicit_period=on  period=ts  equ=P=C  opselect=C  inp2=PCIN>>17  opr=+  inp1=P  carry=CIN  dbl_ovrd=off  block_type=constant
  wx_6 : xbsIndex_r4/Constant  const=wx(6)  gui_display_data_type=Fixed-point  arith_type=Unsigned  n_bits=nbCoord  bin_pt=bpCoord  preci_type=Single  exp_width=8  frac_width=24  explicit_period=on  period=ts  equ=P=C  opselect=C  inp2=PCIN>>17  opr=+  inp1=P  carry=CIN  dbl_ovrd=off  block_type=constant
  wx_7 : xbsIndex_r4/Constant  const=wx(7)  gui_display_data_type=Fixed-point  arith_type=Unsigned  n_bits=nbCoord  bin_pt=bpCoord  preci_type=Single  exp_width=8  frac_width=24  explicit_period=on  period=ts  equ=P=C  opselect=C  inp2=PCIN>>17  opr=+  inp1=P  carry=CIN  dbl_ovrd=off  block_type=constant
  wx_8 : xbsIndex_r4/Constant  const=wx(8)  gui_display_data_type=Fixed-point  arith_type=Unsigned  n_bits=nbCoord  bin_pt=bpCoord  preci_type=Single  exp_width=8  frac_width=24  explicit_period=on  period=ts  equ=P=C  opselect=C  inp2=PCIN>>17  opr=+  inp1=P  carry=CIN  dbl_ovrd=off  block_type=constant
  wx_9 : xbsIndex_r4/Constant  const=wx(9)  gui_display_data_type=Fixed-point  arith_type=Unsigned  n_bits=nbCoord  bin_pt=bpCoord  preci_type=Single  exp_width=8  frac_width=24  explicit_period=on  period=ts  equ=P=C  opselect=C  inp2=PCIN>>17  opr=+  inp1=P  carry=CIN  dbl_ovrd=off  block_type=constant
  wy_1 : xbsIndex_r4/Constant  const=wy(1)  gui_display_data_type=Fixed-point  arith_type=Unsigned  n_bits=nbCoord  bin_pt=bpCoord  preci_type=Single  exp_width=8  frac_width=24  explicit_period=on  period=ts  equ=P=C  opselect=C  inp2=PCIN>>17  opr=+  inp1=P  carry=CIN  dbl_ovrd=off  block_type=constant
  wy_10 : xbsIndex_r4/Constant  const=wy(10)  gui_display_data_type=Fixed-point  arith_type=Unsigned  n_bits=nbCoord  bin_pt=bpCoord  preci_type=Single  exp_width=8  frac_width=24  explicit_period=on  period=ts  equ=P=C  opselect=C  inp2=PCIN>>17  opr=+  inp1=P  carry=CIN  dbl_ovrd=off  block_type=constant
  wy_11 : xbsIndex_r4/Constant  const=wy(11)  gui_display_data_type=Fixed-point  arith_type=Unsigned  n_bits=nbCoord  bin_pt=bpCoord  preci_type=Single  exp_width=8  frac_width=24  explicit_period=on  period=ts  equ=P=C  opselect=C  inp2=PCIN>>17  opr=+  inp1=P  carry=CIN  dbl_ovrd=off  block_type=constant
  wy_12 : xbsIndex_r4/Constant  const=wy(12)  gui_display_data_type=Fixed-point  arith_type=Unsigned  n_bits=nbCoord  bin_pt=bpCoord  preci_type=Single  exp_width=8  frac_width=24  explicit_period=on  period=ts  equ=P=C  opselect=C  inp2=PCIN>>17  opr=+  inp1=P  carry=CIN  dbl_ovrd=off  block_type=constant
  wy_13 : xbsIndex_r4/Constant  const=wy(13)  gui_display_data_type=Fixed-point  arith_type=Unsigned  n_bits=nbCoord  bin_pt=bpCoord  preci_type=Single  exp_width=8  frac_width=24  explicit_period=on  period=ts  equ=P=C  opselect=C  inp2=PCIN>>17  opr=+  inp1=P  carry=CIN  dbl_ovrd=off  block_type=constant
  wy_14 : xbsIndex_r4/Constant  const=wy(14)  gui_display_data_type=Fixed-point  arith_type=Unsigned  n_bits=nbCoord  bin_pt=bpCoord  preci_type=Single  exp_width=8  frac_width=24  explicit_period=on  period=ts  equ=P=C  opselect=C  inp2=PCIN>>17  opr=+  inp1=P  carry=CIN  dbl_ovrd=off  block_type=constant
  wy_15 : xbsIndex_r4/Constant  const=wy(15)  gui_display_data_type=Fixed-point  arith_type=Unsigned  n_bits=nbCoord  bin_pt=bpCoord  preci_type=Single  exp_width=8  frac_width=24  explicit_period=on  period=ts  equ=P=C  opselect=C  inp2=PCIN>>17  opr=+  inp1=P  carry=CIN  dbl_ovrd=off  block_type=constant
  wy_16 : xbsIndex_r4/Constant  const=wy(16)  gui_display_data_type=Fixed-point  arith_type=Unsigned  n_bits=nbCoord  bin_pt=bpCoord  preci_type=Single  exp_width=8  frac_width=24  explicit_period=on  period=ts  equ=P=C  opselect=C  inp2=PCIN>>17  opr=+  inp1=P  carry=CIN  dbl_ovrd=off  block_type=constant
  wy_17 : xbsIndex_r4/Constant  const=wy(17)  gui_display_data_type=Fixed-point  arith_type=Unsigned  n_bits=nbCoord  bin_pt=bpCoord  preci_type=Single  exp_width=8  frac_width=24  explicit_period=on  period=ts  equ=P=C  opselect=C  inp2=PCIN>>17  opr=+  inp1=P  carry=CIN  dbl_ovrd=off  block_type=constant
  wy_18 : xbsIndex_r4/Constant  const=wy(18)  gui_display_data_type=Fixed-point  arith_type=Unsigned  n_bits=nbCoord  bin_pt=bpCoord  preci_type=Single  exp_width=8  frac_width=24  explicit_period=on  period=ts  equ=P=C  opselect=C  inp2=PCIN>>17  opr=+  inp1=P  carry=CIN  dbl_ovrd=off  block_type=constant
  wy_{19,26,35,42} (4 alike) : xbsIndex_r4/Constant  const=wy(19)  gui_display_data_type=Fixed-point  arith_type=Unsigned  n_bits=nbCoord  bin_pt=bpCoord  preci_type=Single  exp_width=8  frac_width=24  explicit_period=on  period=ts  equ=P=C  opselect=C  inp2=PCIN>>17  opr=+  inp1=P  carry=CIN  dbl_ovrd=off  block_type=constant
  wy_2 : xbsIndex_r4/Constant  const=wy(2)  gui_display_data_type=Fixed-point  arith_type=Unsigned  n_bits=nbCoord  bin_pt=bpCoord  preci_type=Single  exp_width=8  frac_width=24  explicit_period=on  period=ts  equ=P=C  opselect=C  inp2=PCIN>>17  opr=+  inp1=P  carry=CIN  dbl_ovrd=off  block_type=constant
  wy_{20,27,36,43} (4 alike) : xbsIndex_r4/Constant  const=wy(20)  gui_display_data_type=Fixed-point  arith_type=Unsigned  n_bits=nbCoord  bin_pt=bpCoord  preci_type=Single  exp_width=8  frac_width=24  explicit_period=on  period=ts  equ=P=C  opselect=C  inp2=PCIN>>17  opr=+  inp1=P  carry=CIN  dbl_ovrd=off  block_type=constant
  wy_{21,28,37,44} (4 alike) : xbsIndex_r4/Constant  const=wy(21)  gui_display_data_type=Fixed-point  arith_type=Unsigned  n_bits=nbCoord  bin_pt=bpCoord  preci_type=Single  exp_width=8  frac_width=24  explicit_period=on  period=ts  equ=P=C  opselect=C  inp2=PCIN>>17  opr=+  inp1=P  carry=CIN  dbl_ovrd=off  block_type=constant
  wy_{22,29,38,45} (4 alike) : xbsIndex_r4/Constant  const=wy(22)  gui_display_data_type=Fixed-point  arith_type=Unsigned  n_bits=nbCoord  bin_pt=bpCoord  preci_type=Single  exp_width=8  frac_width=24  explicit_period=on  period=ts  equ=P=C  opselect=C  inp2=PCIN>>17  opr=+  inp1=P  carry=CIN  dbl_ovrd=off  block_type=constant
  wy_{23,30,39,46} (4 alike) : xbsIndex_r4/Constant  const=wy(23)  gui_display_data_type=Fixed-point  arith_type=Unsigned  n_bits=nbCoord  bin_pt=bpCoord  preci_type=Single  exp_width=8  frac_width=24  explicit_period=on  period=ts  equ=P=C  opselect=C  inp2=PCIN>>17  opr=+  inp1=P  carry=CIN  dbl_ovrd=off  block_type=constant
  wy_{24,31,40,47} (4 alike) : xbsIndex_r4/Constant  const=wy(24)  gui_display_data_type=Fixed-point  arith_type=Unsigned  n_bits=nbCoord  bin_pt=bpCoord  preci_type=Single  exp_width=8  frac_width=24  explicit_period=on  period=ts  equ=P=C  opselect=C  inp2=PCIN>>17  opr=+  inp1=P  carry=CIN  dbl_ovrd=off  block_type=constant
  wy_{25,32,41,48} (4 alike) : xbsIndex_r4/Constant  const=wy(25)  gui_display_data_type=Fixed-point  arith_type=Unsigned  n_bits=nbCoord  bin_pt=bpCoord  preci_type=Single  exp_width=8  frac_width=24  explicit_period=on  period=ts  equ=P=C  opselect=C  inp2=PCIN>>17  opr=+  inp1=P  carry=CIN  dbl_ovrd=off  block_type=constant
  wy_3 : xbsIndex_r4/Constant  const=wy(3)  gui_display_data_type=Fixed-point  arith_type=Unsigned  n_bits=nbCoord  bin_pt=bpCoord  preci_type=Single  exp_width=8  frac_width=24  explicit_period=on  period=ts  equ=P=C  opselect=C  inp2=PCIN>>17  opr=+  inp1=P  carry=CIN  dbl_ovrd=off  block_type=constant
  wy_33 : xbsIndex_r4/Constant  const=wy(17)  gui_display_data_type=Fixed-point  arith_type=Unsigned  n_bits=nbCoord  bin_pt=bpCoord  preci_type=Single  exp_width=8  frac_width=24  explicit_period=on  period=ts  equ=P=C  opselect=C  inp2=PCIN>>17  opr=+  inp1=P  carry=CIN  dbl_ovrd=off  block_type=constant
  wy_34 : xbsIndex_r4/Constant  const=wy(18)  gui_display_data_type=Fixed-point  arith_type=Unsigned  n_bits=nbCoord  bin_pt=bpCoord  preci_type=Single  exp_width=8  frac_width=24  explicit_period=on  period=ts  equ=P=C  opselect=C  inp2=PCIN>>17  opr=+  inp1=P  carry=CIN  dbl_ovrd=off  block_type=constant
  wy_4 : xbsIndex_r4/Constant  const=wy(4)  gui_display_data_type=Fixed-point  arith_type=Unsigned  n_bits=nbCoord  bin_pt=bpCoord  preci_type=Single  exp_width=8  frac_width=24  explicit_period=on  period=ts  equ=P=C  opselect=C  inp2=PCIN>>17  opr=+  inp1=P  carry=CIN  dbl_ovrd=off  block_type=constant
  wy_49 : xbsIndex_r4/Constant  const=wy(17)  gui_display_data_type=Fixed-point  arith_type=Unsigned  n_bits=nbCoord  bin_pt=bpCoord  preci_type=Single  exp_width=8  frac_width=24  explicit_period=on  period=ts  equ=P=C  opselect=C  inp2=PCIN>>17  opr=+  inp1=P  carry=CIN  dbl_ovrd=off  block_type=constant
  wy_5 : xbsIndex_r4/Constant  const=wy(5)  gui_display_data_type=Fixed-point  arith_type=Unsigned  n_bits=nbCoord  bin_pt=bpCoord  preci_type=Single  exp_width=8  frac_width=24  explicit_period=on  period=ts  equ=P=C  opselect=C  inp2=PCIN>>17  opr=+  inp1=P  carry=CIN  dbl_ovrd=off  block_type=constant
  wy_6 : xbsIndex_r4/Constant  const=wy(6)  gui_display_data_type=Fixed-point  arith_type=Unsigned  n_bits=nbCoord  bin_pt=bpCoord  preci_type=Single  exp_width=8  frac_width=24  explicit_period=on  period=ts  equ=P=C  opselect=C  inp2=PCIN>>17  opr=+  inp1=P  carry=CIN  dbl_ovrd=off  block_type=constant
  wy_7 : xbsIndex_r4/Constant  const=wy(7)  gui_display_data_type=Fixed-point  arith_type=Unsigned  n_bits=nbCoord  bin_pt=bpCoord  preci_type=Single  exp_width=8  frac_width=24  explicit_period=on  period=ts  equ=P=C  opselect=C  inp2=PCIN>>17  opr=+  inp1=P  carry=CIN  dbl_ovrd=off  block_type=constant
  wy_8 : xbsIndex_r4/Constant  const=wy(8)  gui_display_data_type=Fixed-point  arith_type=Unsigned  n_bits=nbCoord  bin_pt=bpCoord  preci_type=Single  exp_width=8  frac_width=24  explicit_period=on  period=ts  equ=P=C  opselect=C  inp2=PCIN>>17  opr=+  inp1=P  carry=CIN  dbl_ovrd=off  block_type=constant
  wy_9 : xbsIndex_r4/Constant  const=wy(9)  gui_display_data_type=Fixed-point  arith_type=Unsigned  n_bits=nbCoord  bin_pt=bpCoord  preci_type=Single  exp_width=8  frac_width=24  explicit_period=on  period=ts  equ=P=C  opselect=C  inp2=PCIN>>17  opr=+  inp1=P  carry=CIN  dbl_ovrd=off  block_type=constant
  wx1 : Outport
  wy1 : Outport  Port=2
  wx2 : Outport  Port=3
  wy2 : Outport  Port=4
  wx3 : Outport  Port=5
  wy3 : Outport  Port=6
  wx4 : Outport  Port=7
  wy4 : Outport  Port=8
  wx5 : Outport  Port=9
  wy5 : Outport  Port=10
  wx6 : Outport  Port=11
  wy6 : Outport  Port=12
  wx7 : Outport  Port=13
  wy7 : Outport  Port=14
  wx8 : Outport  Port=15
  wy8 : Outport  Port=16
  wx9 : Outport  Port=17
  wy9 : Outport  Port=18
  wx10 : Outport  Port=19
  wy10 : Outport  Port=20
  wx11 : Outport  Port=21
  wy11 : Outport  Port=22
  wx12 : Outport  Port=23
  wy12 : Outport  Port=24
  wx13 : Outport  Port=25
  wy13 : Outport  Port=26
  wx14 : Outport  Port=27
  wy14 : Outport  Port=28
  wx15 : Outport  Port=29
  wy15 : Outport  Port=30
  wx16 : Outport  Port=31
  wy16 : Outport  Port=32
  wx17 : Outport  Port=33
  wy17 : Outport  Port=34
  wx18 : Outport  Port=35
  wy18 : Outport  Port=36
  wx19 : Outport  Port=37
  wy19 : Outport  Port=38
  wx20 : Outport  Port=39
  wy20 : Outport  Port=40
  wx21 : Outport  Port=41
  wy21 : Outport  Port=42
  wx22 : Outport  Port=43
  wy22 : Outport  Port=44
  wx23 : Outport  Port=45
  wy23 : Outport  Port=46
  wx24 : Outport  Port=47
  wy24 : Outport  Port=48
  wx25 : Outport  Port=49
  wy25 : Outport  Port=50
  wx26 : Outport  Port=51
  wy26 : Outport  Port=52
  wx27 : Outport  Port=53
  wy27 : Outport  Port=54
  wx28 : Outport  Port=55
  wy28 : Outport  Port=56
  wx29 : Outport  Port=57
  wy29 : Outport  Port=58
  wx30 : Outport  Port=59
  wy30 : Outport  Port=60
  wx31 : Outport  Port=61
  wy31 : Outport  Port=62
  wx32 : Outport  Port=63
  wy32 : Outport  Port=64
  wx33 : Outport  Port=65
  wy33 : Outport  Port=66
  wx34 : Outport  Port=67
  wy34 : Outport  Port=68
  wx35 : Outport  Port=69
  wy35 : Outport  Port=70
  wx36 : Outport  Port=71
  wy36 : Outport  Port=72
  wx37 : Outport  Port=73
  wy37 : Outport  Port=74
  wx38 : Outport  Port=75
  wy38 : Outport  Port=76
  wx39 : Outport  Port=77
  wy39 : Outport  Port=78
  wx40 : Outport  Port=79
  wy40 : Outport  Port=80
  wx41 : Outport  Port=81
  wy41 : Outport  Port=82
  wx42 : Outport  Port=83
  wy42 : Outport  Port=84
  wx43 : Outport  Port=85
  wy43 : Outport  Port=86
  wx44 : Outport  Port=87
  wy44 : Outport  Port=88
  wx45 : Outport  Port=89
  wy45 : Outport  Port=90
  wx46 : Outport  Port=91
  wy46 : Outport  Port=92
  wx47 : Outport  Port=93
  wy47 : Outport  Port=94
  wx48 : Outport  Port=95
  wy48 : Outport  Port=96
  wx49 : Outport  Port=97
  wy49 : Outport  Port=98
  wires:
  wy_2/1 -> wy2/1
  wy_16/1 -> wy16/1
  wx_9/1 -> wx9/1
  wy_3/1 -> wy3/1
  wx_3/1 -> wx3/1
  wy_5/1 -> wy5/1
  wx_2/1 -> wx2/1
  wx_12/1 -> wx12/1
  wy_6/1 -> wy6/1
  wx_11/1 -> wx11/1
  wy_11/1 -> wy11/1
  wy_14/1 -> wy14/1
  wy_8/1 -> wy8/1
  wy_7/1 -> wy7/1
  wx_8/1 -> wx8/1
  wx_5/1 -> wx5/1
  wx_4/1 -> wx4/1
  wx_7/1 -> wx7/1
  wx_15/1 -> wx15/1
  wy_1/1 -> wy1/1
  wy_4/1 -> wy4/1
  wx_16/1 -> wx16/1
  wx_6/1 -> wx6/1
  wy_13/1 -> wy13/1
  wx_14/1 -> wx14/1
  wy_15/1 -> wy15/1
  wx_10/1 -> wx10/1
  wy_10/1 -> wy10/1
  wx_13/1 -> wx13/1
  wy_9/1 -> wy9/1
  wy_12/1 -> wy12/1
  wy_25/1 -> wy25/1
  wx_18/1 -> wx18/1
  wx_21/1 -> wx21/1
  wx_20/1 -> wx20/1
  wy_20/1 -> wy20/1
  wy_23/1 -> wy23/1
  wy_17/1 -> wy17/1
  wx_17/1 -> wx17/1
  wx_24/1 -> wx24/1
  wx_25/1 -> wx25/1
  wy_22/1 -> wy22/1
  wx_23/1 -> wx23/1
  wy_24/1 -> wy24/1
  wx_19/1 -> wx19/1
  wy_19/1 -> wy19/1
  wx_22/1 -> wx22/1
  wy_18/1 -> wy18/1
  wy_21/1 -> wy21/1
  wx_1/1 -> wx1/1
  wy_32/1 -> wy32/1
  wx_28/1 -> wx28/1
  wx_27/1 -> wx27/1
  wy_27/1 -> wy27/1
  wy_30/1 -> wy30/1
  wx_31/1 -> wx31/1
  wx_32/1 -> wx32/1
  wy_29/1 -> wy29/1
  wx_30/1 -> wx30/1
  wy_31/1 -> wy31/1
  wx_26/1 -> wx26/1
  wy_26/1 -> wy26/1
  wx_29/1 -> wx29/1
  wy_28/1 -> wy28/1
  wy_41/1 -> wy41/1
  wx_34/1 -> wx34/1
  wx_37/1 -> wx37/1
  wx_36/1 -> wx36/1
  wy_36/1 -> wy36/1
  wy_39/1 -> wy39/1
  wy_33/1 -> wy33/1
  wx_33/1 -> wx33/1
  wx_40/1 -> wx40/1
  wx_41/1 -> wx41/1
  wy_38/1 -> wy38/1
  wx_39/1 -> wx39/1
  wy_40/1 -> wy40/1
  wx_35/1 -> wx35/1
  wy_35/1 -> wy35/1
  wx_38/1 -> wx38/1
  wy_34/1 -> wy34/1
  wy_37/1 -> wy37/1
  wy_48/1 -> wy48/1
  wx_44/1 -> wx44/1
  wx_43/1 -> wx43/1
  wy_43/1 -> wy43/1
  wy_46/1 -> wy46/1
  wx_47/1 -> wx47/1
  wx_48/1 -> wx48/1
  wy_45/1 -> wy45/1
  wx_46/1 -> wx46/1
  wy_47/1 -> wy47/1
  wx_42/1 -> wx42/1
  wy_42/1 -> wy42/1
  wx_45/1 -> wx45/1
  wy_44/1 -> wy44/1
  wy_49/1 -> wy49/1
  wx_49/1 -> wx49/1
